simulink model "sm_import_stewart_platform"  (R2021b)
settings: Solver=ode45  StartTime=0.0  StopTime=10.0  RelTol=1e-3  EnableMultiTasking=on
model workspace (MATLAB code in the model file):
  | % The six origin vectors correspond to the six legs of the Stewart platform
  | stewart_pos_base = [0.0962 0 -0.0336; 0.0772 0 -0.0665;-0.0742 0 -0.0599;...
  |     -0.0962 0 -0.0336; -0.0190 0 0.1001;0.019 0 0.1001];
  | 
  | % Corresponding body points on the top plate
  | stewart_body_pts = [0.0607 0 0.0203; 0.0128 0 -0.0628; -0.0145 0 -0.0669; ...
  |     -0.0652 0 0.0208; -0.0507 0 0.046; 0.0507 0 0.046]';
  | 
  | % Leg length
  | leg_length = 0.19*ones(1,6);
undefined symbols (not defined in the file): X, Y, Z
libraries: sm_lib x1374, nesl_utility x19
(part 16 of 28)

== system sm_import_stewart_platform/Stewart Platform/Imported Stewart Platform/ActuatorAssm1_2/CarrierAssm_1_RIGID/HR_1_Motor_1_RIGID ==
  ReferenceFrame : sm_lib/Frames and Transforms/Reference Frame
  Solid : sm_lib/Body Elements/File Solid  ExtGeomFileName=HR_1_Motor_Default_sldprt.STL  UnitType=Custom  ExtGeomFileUnits=cm  StepReaderType=HEX  ExportConvexHullGeometry=off  InertiaType=Custom  Mass=0.016323277951690116  MassUnits=kg  CenterOfMass=[1.1461762495150611 1.9087990143138187 0.39999826480475109]  CenterOfMassUnits=cm  MomentsOfInertia=[0.022976248526302246 0.016967187564536409 0.038272540312041692]  MomentsOfInertiaUnits=kg*cm^2  ProductsOfInertia=[-6.3449814973716521e-08 -1.4415405966206584e-07 -0.0031628803180496112]  ProductsOfInertiaUnits=kg*cm^2  BasedOnType=Density  Density=1000  DensityUnits=kg/(m^3)  DoExposeReferenceFrame=on  SerializedFrames=<Frames/>  GraphicType=FromGeometry  MarkerShape=Sphere  MarkerSize=10  MarkerSizeUnits=m  GraphicVisPropType=SimpleVisualProperties  GraphicDiffuseColor=[0.95999999999999996 0.69647058823529406 0.56847058823529406]  GraphicSpecularColor=[0.5 0.5 0.5 1.0]  GraphicAmbientColor=[0.15 0.15 0.15 1.0]  GraphicEmissiveColor=[0.0 0.0 0.0 1.0]  GraphicShininess=75  GraphicOpacity=1
  F : PMIOPort  Side=Left
  connections:
  ReferenceFrame/RConn1 -- Solid/RConn1 -- F/RConn1

== system sm_import_stewart_platform/Stewart Platform/Imported Stewart Platform/ActuatorAssm1_2/CarrierAssm_1_RIGID/HR_1_Motor_2_RIGID ==
  ReferenceFrame : sm_lib/Frames and Transforms/Reference Frame
  Solid : sm_lib/Body Elements/File Solid  ExtGeomFileName=HR_1_Motor_Default_sldprt.STL  UnitType=Custom  ExtGeomFileUnits=cm  StepReaderType=HEX  ExportConvexHullGeometry=off  InertiaType=Custom  Mass=0.016323277951690116  MassUnits=kg  CenterOfMass=[1.1461762495150611 1.9087990143138187 0.39999826480475109]  CenterOfMassUnits=cm  MomentsOfInertia=[0.022976248526302246 0.016967187564536409 0.038272540312041692]  MomentsOfInertiaUnits=kg*cm^2  ProductsOfInertia=[-6.3449814973716521e-08 -1.4415405966206584e-07 -0.0031628803180496112]  ProductsOfInertiaUnits=kg*cm^2  BasedOnType=Density  Density=1000  DensityUnits=kg/(m^3)  DoExposeReferenceFrame=on  SerializedFrames=<Frames/>  GraphicType=FromGeometry  MarkerShape=Sphere  MarkerSize=10  MarkerSizeUnits=m  GraphicVisPropType=SimpleVisualProperties  GraphicDiffuseColor=[0.95999999999999996 0.69647058823529406 0.56847058823529406]  GraphicSpecularColor=[0.5 0.5 0.5 1.0]  GraphicAmbientColor=[0.15 0.15 0.15 1.0]  GraphicEmissiveColor=[0.0 0.0 0.0 1.0]  GraphicShininess=75  GraphicOpacity=1
  F : PMIOPort  Side=Left
  connections:
  ReferenceFrame/RConn1 -- Solid/RConn1 -- F/RConn1

== system sm_import_stewart_platform/Stewart Platform/Imported Stewart Platform/ActuatorAssm1_2/CarrierAssm_1_RIGID/Hexagon_Socket_Button_Head_Screw_M3x6_1_RIGID ==
  ReferenceFrame : sm_lib/Frames and Transforms/Reference Frame
  Solid : sm_lib/Body Elements/File Solid  ExtGeomFileName=Hexagon_Socket_Button_Head_Screw_M3x6_Default_sldprt.STL  UnitType=Custom  ExtGeomFileUnits=cm  StepReaderType=HEX  ExportConvexHullGeometry=off  InertiaType=Custom  Mass=0.00056348185373580135  MassUnits=kg  CenterOfMass=[0.14356282026314221 8.1476592298985412e-06 5.8788316934839061e-08]  CenterOfMassUnits=cm  MomentsOfInertia=[1.3098988700385332e-05 3.5078394083955334e-05 3.5077439490752727e-05]  MomentsOfInertiaUnits=kg*cm^2  ProductsOfInertia=[-6.7519077190030419e-11 7.6873810692743504e-12 1.0654186206953444e-09]  ProductsOfInertiaUnits=kg*cm^2  BasedOnType=Density  Density=1000  DensityUnits=kg/(m^3)  DoExposeReferenceFrame=on  SerializedFrames=<Frames/>  GraphicType=FromGeometry  MarkerShape=Sphere  MarkerSize=10  MarkerSizeUnits=m  GraphicVisPropType=SimpleVisualProperties  GraphicDiffuseColor=[0.72282352941176464 0.72282352941176464 0.72282352941176464]  GraphicSpecularColor=[0.5 0.5 0.5 1.0]  GraphicAmbientColor=[0.15 0.15 0.15 1.0]  GraphicEmissiveColor=[0.0 0.0 0.0 1.0]  GraphicShininess=75  GraphicOpacity=1
  F : PMIOPort  Side=Left
  connections:
  ReferenceFrame/RConn1 -- Solid/RConn1 -- F/RConn1

== system sm_import_stewart_platform/Stewart Platform/Imported Stewart Platform/ActuatorAssm1_2/CarrierAssm_1_RIGID/Hexagon_Socket_Button_Head_Screw_M3x6_2_RIGID ==
  ReferenceFrame : sm_lib/Frames and Transforms/Reference Frame
  Solid : sm_lib/Body Elements/File Solid  ExtGeomFileName=Hexagon_Socket_Button_Head_Screw_M3x6_Default_sldprt.STL  UnitType=Custom  ExtGeomFileUnits=cm  StepReaderType=HEX  ExportConvexHullGeometry=off  InertiaType=Custom  Mass=0.00056348185373580135  MassUnits=kg  CenterOfMass=[0.14356282026314221 8.1476592298985412e-06 5.8788316934839061e-08]  CenterOfMassUnits=cm  MomentsOfInertia=[1.3098988700385332e-05 3.5078394083955334e-05 3.5077439490752727e-05]  MomentsOfInertiaUnits=kg*cm^2  ProductsOfInertia=[-6.7519077190030419e-11 7.6873810692743504e-12 1.0654186206953444e-09]  ProductsOfInertiaUnits=kg*cm^2  BasedOnType=Density  Density=1000  DensityUnits=kg/(m^3)  DoExposeReferenceFrame=on  SerializedFrames=<Frames/>  GraphicType=FromGeometry  MarkerShape=Sphere  MarkerSize=10  MarkerSizeUnits=m  GraphicVisPropType=SimpleVisualProperties  GraphicDiffuseColor=[0.72282352941176464 0.72282352941176464 0.72282352941176464]  GraphicSpecularColor=[0.5 0.5 0.5 1.0]  GraphicAmbientColor=[0.15 0.15 0.15 1.0]  GraphicEmissiveColor=[0.0 0.0 0.0 1.0]  GraphicShininess=75  GraphicOpacity=1
  F : PMIOPort  Side=Left
  connections:
  ReferenceFrame/RConn1 -- Solid/RConn1 -- F/RConn1

== system sm_import_stewart_platform/Stewart Platform/Imported Stewart Platform/ActuatorAssm1_2/CarrierAssm_1_RIGID/Hexagon_Socket_Button_Head_Screw_M3x6_3_RIGID ==
  ReferenceFrame : sm_lib/Frames and Transforms/Reference Frame
  Solid : sm_lib/Body Elements/File Solid  ExtGeomFileName=Hexagon_Socket_Button_Head_Screw_M3x6_Default_sldprt.STL  UnitType=Custom  ExtGeomFileUnits=cm  StepReaderType=HEX  ExportConvexHullGeometry=off  InertiaType=Custom  Mass=0.00056348185373580135  MassUnits=kg  CenterOfMass=[0.14356282026314221 8.1476592298985412e-06 5.8788316934839061e-08]  CenterOfMassUnits=cm  MomentsOfInertia=[1.3098988700385332e-05 3.5078394083955334e-05 3.5077439490752727e-05]  MomentsOfInertiaUnits=kg*cm^2  ProductsOfInertia=[-6.7519077190030419e-11 7.6873810692743504e-12 1.0654186206953444e-09]  ProductsOfInertiaUnits=kg*cm^2  BasedOnType=Density  Density=1000  DensityUnits=kg/(m^3)  DoExposeReferenceFrame=on  SerializedFrames=<Frames/>  GraphicType=FromGeometry  MarkerShape=Sphere  MarkerSize=10  MarkerSizeUnits=m  GraphicVisPropType=SimpleVisualProperties  GraphicDiffuseColor=[0.72282352941176464 0.72282352941176464 0.72282352941176464]  GraphicSpecularColor=[0.5 0.5 0.5 1.0]  GraphicAmbientColor=[0.15 0.15 0.15 1.0]  GraphicEmissiveColor=[0.0 0.0 0.0 1.0]  GraphicShininess=75  GraphicOpacity=1
  F : PMIOPort  Side=Left
  connections:
  ReferenceFrame/RConn1 -- Solid/RConn1 -- F/RConn1

== system sm_import_stewart_platform/Stewart Platform/Imported Stewart Platform/ActuatorAssm1_2/CarrierAssm_1_RIGID/Hexagon_Socket_Button_Head_Screw_M3x6_4_RIGID ==
  ReferenceFrame : sm_lib/Frames and Transforms/Reference Frame
  Solid : sm_lib/Body Elements/File Solid  ExtGeomFileName=Hexagon_Socket_Button_Head_Screw_M3x6_Default_sldprt.STL  UnitType=Custom  ExtGeomFileUnits=cm  StepReaderType=HEX  ExportConvexHullGeometry=off  InertiaType=Custom  Mass=0.00056348185373580135  MassUnits=kg  CenterOfMass=[0.14356282026314221 8.1476592298985412e-06 5.8788316934839061e-08]  CenterOfMassUnits=cm  MomentsOfInertia=[1.3098988700385332e-05 3.5078394083955334e-05 3.5077439490752727e-05]  MomentsOfInertiaUnits=kg*cm^2  ProductsOfInertia=[-6.7519077190030419e-11 7.6873810692743504e-12 1.0654186206953444e-09]  ProductsOfInertiaUnits=kg*cm^2  BasedOnType=Density  Density=1000  DensityUnits=kg/(m^3)  DoExposeReferenceFrame=on  SerializedFrames=<Frames/>  GraphicType=FromGeometry  MarkerShape=Sphere  MarkerSize=10  MarkerSizeUnits=m  GraphicVisPropType=SimpleVisualProperties  GraphicDiffuseColor=[0.72282352941176464 0.72282352941176464 0.72282352941176464]  GraphicSpecularColor=[0.5 0.5 0.5 1.0]  GraphicAmbientColor=[0.15 0.15 0.15 1.0]  GraphicEmissiveColor=[0.0 0.0 0.0 1.0]  GraphicShininess=75  GraphicOpacity=1
  F : PMIOPort  Side=Left
  connections:
  ReferenceFrame/RConn1 -- Solid/RConn1 -- F/RConn1

== system sm_import_stewart_platform/Stewart Platform/Imported Stewart Platform/ActuatorAssm1_2/CarrierAssm_1_RIGID/Hexagon_Socket_Button_Head_Screw_M3x6_5_RIGID ==
  ReferenceFrame : sm_lib/Frames and Transforms/Reference Frame
  Solid : sm_lib/Body Elements/File Solid  ExtGeomFileName=Hexagon_Socket_Button_Head_Screw_M3x6_Default_sldprt.STL  UnitType=Custom  ExtGeomFileUnits=cm  StepReaderType=HEX  ExportConvexHullGeometry=off  InertiaType=Custom  Mass=0.00056348185373580135  MassUnits=kg  CenterOfMass=[0.14356282026314221 8.1476592298985412e-06 5.8788316934839061e-08]  CenterOfMassUnits=cm  MomentsOfInertia=[1.3098988700385332e-05 3.5078394083955334e-05 3.5077439490752727e-05]  MomentsOfInertiaUnits=kg*cm^2  ProductsOfInertia=[-6.7519077190030419e-11 7.6873810692743504e-12 1.0654186206953444e-09]  ProductsOfInertiaUnits=kg*cm^2  BasedOnType=Density  Density=1000  DensityUnits=kg/(m^3)  DoExposeReferenceFrame=on  SerializedFrames=<Frames/>  GraphicType=FromGeometry  MarkerShape=Sphere  MarkerSize=10  MarkerSizeUnits=m  GraphicVisPropType=SimpleVisualProperties  GraphicDiffuseColor=[0.72282352941176464 0.72282352941176464 0.72282352941176464]  GraphicSpecularColor=[0.5 0.5 0.5 1.0]  GraphicAmbientColor=[0.15 0.15 0.15 1.0]  GraphicEmissiveColor=[0.0 0.0 0.0 1.0]  GraphicShininess=75  GraphicOpacity=1
  F : PMIOPort  Side=Left
  connections:
  ReferenceFrame/RConn1 -- Solid/RConn1 -- F/RConn1

== system sm_import_stewart_platform/Stewart Platform/Imported Stewart Platform/ActuatorAssm1_2/CarrierAssm_1_RIGID/Hexagon_Socket_Button_Head_Screw_M3x6_6_RIGID ==
  ReferenceFrame : sm_lib/Frames and Transforms/Reference Frame
  Solid : sm_lib/Body Elements/File Solid  ExtGeomFileName=Hexagon_Socket_Button_Head_Screw_M3x6_Default_sldprt.STL  UnitType=Custom  ExtGeomFileUnits=cm  StepReaderType=HEX  ExportConvexHullGeometry=off  InertiaType=Custom  Mass=0.00056348185373580135  MassUnits=kg  CenterOfMass=[0.14356282026314221 8.1476592298985412e-06 5.8788316934839061e-08]  CenterOfMassUnits=cm  MomentsOfInertia=[1.3098988700385332e-05 3.5078394083955334e-05 3.5077439490752727e-05]  MomentsOfInertiaUnits=kg*cm^2  ProductsOfInertia=[-6.7519077190030419e-11 7.6873810692743504e-12 1.0654186206953444e-09]  ProductsOfInertiaUnits=kg*cm^2  BasedOnType=Density  Density=1000  DensityUnits=kg/(m^3)  DoExposeReferenceFrame=on  SerializedFrames=<Frames/>  GraphicType=FromGeometry  MarkerShape=Sphere  MarkerSize=10  MarkerSizeUnits=m  GraphicVisPropType=SimpleVisualProperties  GraphicDiffuseColor=[0.72282352941176464 0.72282352941176464 0.72282352941176464]  GraphicSpecularColor=[0.5 0.5 0.5 1.0]  GraphicAmbientColor=[0.15 0.15 0.15 1.0]  GraphicEmissiveColor=[0.0 0.0 0.0 1.0]  GraphicShininess=75  GraphicOpacity=1
  F : PMIOPort  Side=Left
  connections:
  ReferenceFrame/RConn1 -- Solid/RConn1 -- F/RConn1

== system sm_import_stewart_platform/Stewart Platform/Imported Stewart Platform/ActuatorAssm1_2/CarrierAssm_1_RIGID/Hexagon_Socket_Button_Head_Screw_M3x6_7_RIGID ==
  ReferenceFrame : sm_lib/Frames and Transforms/Reference Frame
  Solid : sm_lib/Body Elements/File Solid  ExtGeomFileName=Hexagon_Socket_Button_Head_Screw_M3x6_Default_sldprt.STL  UnitType=Custom  ExtGeomFileUnits=cm  StepReaderType=HEX  ExportConvexHullGeometry=off  InertiaType=Custom  Mass=0.00056348185373580135  MassUnits=kg  CenterOfMass=[0.14356282026314221 8.1476592298985412e-06 5.8788316934839061e-08]  CenterOfMassUnits=cm  MomentsOfInertia=[1.3098988700385332e-05 3.5078394083955334e-05 3.5077439490752727e-05]  MomentsOfInertiaUnits=kg*cm^2  ProductsOfInertia=[-6.7519077190030419e-11 7.6873810692743504e-12 1.0654186206953444e-09]  ProductsOfInertiaUnits=kg*cm^2  BasedOnType=Density  Density=1000  DensityUnits=kg/(m^3)  DoExposeReferenceFrame=on  SerializedFrames=<Frames/>  GraphicType=FromGeometry  MarkerShape=Sphere  MarkerSize=10  MarkerSizeUnits=m  GraphicVisPropType=SimpleVisualProperties  GraphicDiffuseColor=[0.72282352941176464 0.72282352941176464 0.72282352941176464]  GraphicSpecularColor=[0.5 0.5 0.5 1.0]  GraphicAmbientColor=[0.15 0.15 0.15 1.0]  GraphicEmissiveColor=[0.0 0.0 0.0 1.0]  GraphicShininess=75  GraphicOpacity=1
  F : PMIOPort  Side=Left
  connections:
  ReferenceFrame/RConn1 -- Solid/RConn1 -- F/RConn1

== system sm_import_stewart_platform/Stewart Platform/Imported Stewart Platform/ActuatorAssm1_2/CarrierAssm_1_RIGID/Hexagon_Socket_Button_Head_Screw_M3x6_8_RIGID ==
  ReferenceFrame : sm_lib/Frames and Transforms/Reference Frame
  Solid : sm_lib/Body Elements/File Solid  ExtGeomFileName=Hexagon_Socket_Button_Head_Screw_M3x6_Default_sldprt.STL  UnitType=Custom  ExtGeomFileUnits=cm  StepReaderType=HEX  ExportConvexHullGeometry=off  InertiaType=Custom  Mass=0.00056348185373580135  MassUnits=kg  CenterOfMass=[0.14356282026314221 8.1476592298985412e-06 5.8788316934839061e-08]  CenterOfMassUnits=cm  MomentsOfInertia=[1.3098988700385332e-05 3.5078394083955334e-05 3.5077439490752727e-05]  MomentsOfInertiaUnits=kg*cm^2  ProductsOfInertia=[-6.7519077190030419e-11 7.6873810692743504e-12 1.0654186206953444e-09]  ProductsOfInertiaUnits=kg*cm^2  BasedOnType=Density  Density=1000  DensityUnits=kg/(m^3)  DoExposeReferenceFrame=on  SerializedFrames=<Frames/>  GraphicType=FromGeometry  MarkerShape=Sphere  MarkerSize=10  MarkerSizeUnits=m  GraphicVisPropType=SimpleVisualProperties  GraphicDiffuseColor=[0.72282352941176464 0.72282352941176464 0.72282352941176464]  GraphicSpecularColor=[0.5 0.5 0.5 1.0]  GraphicAmbientColor=[0.15 0.15 0.15 1.0]  GraphicEmissiveColor=[0.0 0.0 0.0 1.0]  GraphicShininess=75  GraphicOpacity=1
  F : PMIOPort  Side=Left
  connections:
  ReferenceFrame/RConn1 -- Solid/RConn1 -- F/RConn1

== system sm_import_stewart_platform/Stewart Platform/Imported Stewart Platform/ActuatorAssm1_2/CarrierAssm_1_RIGID/Hexagon_Socket_Head_Cap_Screw_M3x5_1_RIGID ==
  ReferenceFrame : sm_lib/Frames and Transforms/Reference Frame
  Solid : sm_lib/Body Elements/File Solid  ExtGeomFileName=Hexagon_Socket_Head_Cap_Screw_M3x5_Default_sldprt.STL  UnitType=Custom  ExtGeomFileUnits=cm  StepReaderType=HEX  ExportConvexHullGeometry=off  InertiaType=Custom  Mass=0.00075563833672042757  MassUnits=kg  CenterOfMass=[-0.00070356125816108312 3.3976681789998727e-05 2.4288939549848704e-07]  CenterOfMassUnits=cm  MomentsOfInertia=[2.3283103549749918e-05 4.6860987295278262e-05 4.6851281632327237e-05]  MomentsOfInertiaUnits=kg*cm^2  ProductsOfInertia=[-6.6364273820729613e-10 4.0249100574764394e-11 5.6302615064034264e-09]  ProductsOfInertiaUnits=kg*cm^2  BasedOnType=Density  Density=1000  DensityUnits=kg/(m^3)  DoExposeReferenceFrame=on  SerializedFrames=<Frames/>  GraphicType=FromGeometry  MarkerShape=Sphere  MarkerSize=10  MarkerSizeUnits=m  GraphicVisPropType=SimpleVisualProperties  GraphicDiffuseColor=[0.72282352941176464 0.72282352941176464 0.72282352941176464]  GraphicSpecularColor=[0.5 0.5 0.5 1.0]  GraphicAmbientColor=[0.15 0.15 0.15 1.0]  GraphicEmissiveColor=[0.0 0.0 0.0 1.0]  GraphicShininess=75  GraphicOpacity=1
  F : PMIOPort  Side=Left
  connections:
  ReferenceFrame/RConn1 -- Solid/RConn1 -- F/RConn1

== system sm_import_stewart_platform/Stewart Platform/Imported Stewart Platform/ActuatorAssm1_2/CarrierAssm_1_RIGID/Hexagon_Socket_Head_Cap_Screw_M3x5_2_RIGID ==
  ReferenceFrame : sm_lib/Frames and Transforms/Reference Frame
  Solid : sm_lib/Body Elements/File Solid  ExtGeomFileName=Hexagon_Socket_Head_Cap_Screw_M3x5_Default_sldprt.STL  UnitType=Custom  ExtGeomFileUnits=cm  StepReaderType=HEX  ExportConvexHullGeometry=off  InertiaType=Custom  Mass=0.00075563833672042757  MassUnits=kg  CenterOfMass=[-0.00070356125816108312 3.3976681789998727e-05 2.4288939549848704e-07]  CenterOfMassUnits=cm  MomentsOfInertia=[2.3283103549749918e-05 4.6860987295278262e-05 4.6851281632327237e-05]  MomentsOfInertiaUnits=kg*cm^2  ProductsOfInertia=[-6.6364273820729613e-10 4.0249100574764394e-11 5.6302615064034264e-09]  ProductsOfInertiaUnits=kg*cm^2  BasedOnType=Density  Density=1000  DensityUnits=kg/(m^3)  DoExposeReferenceFrame=on  SerializedFrames=<Frames/>  GraphicType=FromGeometry  MarkerShape=Sphere  MarkerSize=10  MarkerSizeUnits=m  GraphicVisPropType=SimpleVisualProperties  GraphicDiffuseColor=[0.72282352941176464 0.72282352941176464 0.72282352941176464]  GraphicSpecularColor=[0.5 0.5 0.5 1.0]  GraphicAmbientColor=[0.15 0.15 0.15 1.0]  GraphicEmissiveColor=[0.0 0.0 0.0 1.0]  GraphicShininess=75  GraphicOpacity=1
  F : PMIOPort  Side=Left
  connections:
  ReferenceFrame/RConn1 -- Solid/RConn1 -- F/RConn1

== system sm_import_stewart_platform/Stewart Platform/Imported Stewart Platform/ActuatorAssm1_2/CarrierAssm_1_RIGID/Hexagon_Socket_Set_Screw_M3x3_1_RIGID ==
  ReferenceFrame : sm_lib/Frames and Transforms/Reference Frame
  Solid : sm_lib/Body Elements/File Solid  ExtGeomFileName=Hexagon_Socket_Set_Screw_M3x3_Default_sldprt.STL  UnitType=Custom  ExtGeomFileUnits=cm  StepReaderType=HEX  ExportConvexHullGeometry=off  InertiaType=Custom  Mass=0.00013414962639699338  MassUnits=kg  CenterOfMass=[0.14346797240988166 0 0]  CenterOfMassUnits=cm  MomentsOfInertia=[1.6122422751910497e-06 1.6862757603444589e-06 1.6862757577761036e-06]  MomentsOfInertiaUnits=kg*cm^2  ProductsOfInertia=[0 0 0]  ProductsOfInertiaUnits=kg*cm^2  BasedOnType=Density  Density=1000  DensityUnits=kg/(m^3)  DoExposeReferenceFrame=on  SerializedFrames=<Frames/>  GraphicType=FromGeometry  MarkerShape=Sphere  MarkerSize=10  MarkerSizeUnits=m  GraphicVisPropType=SimpleVisualProperties  GraphicDiffuseColor=[0.72282352941176464 0.72282352941176464 0.72282352941176464]  GraphicSpecularColor=[0.5 0.5 0.5 1.0]  GraphicAmbientColor=[0.15 0.15 0.15 1.0]  GraphicEmissiveColor=[0.0 0.0 0.0 1.0]  GraphicShininess=75  GraphicOpacity=1
  F : PMIOPort  Side=Left
  connections:
  ReferenceFrame/RConn1 -- Solid/RConn1 -- F/RConn1

== system sm_import_stewart_platform/Stewart Platform/Imported Stewart Platform/ActuatorAssm1_2/CarrierAssm_1_RIGID/Hexagon_Socket_Set_Screw_M3x3_2_RIGID ==
  ReferenceFrame : sm_lib/Frames and Transforms/Reference Frame
  Solid : sm_lib/Body Elements/File Solid  ExtGeomFileName=Hexagon_Socket_Set_Screw_M3x3_Default_sldprt.STL  UnitType=Custom  ExtGeomFileUnits=cm  StepReaderType=HEX  ExportConvexHullGeometry=off  InertiaType=Custom  Mass=0.00013414962639699338  MassUnits=kg  CenterOfMass=[0.14346797240988166 0 0]  CenterOfMassUnits=cm  MomentsOfInertia=[1.6122422751910497e-06 1.6862757603444589e-06 1.6862757577761036e-06]  MomentsOfInertiaUnits=kg*cm^2  ProductsOfInertia=[0 0 0]  ProductsOfInertiaUnits=kg*cm^2  BasedOnType=Density  Density=1000  DensityUnits=kg/(m^3)  DoExposeReferenceFrame=on  SerializedFrames=<Frames/>  GraphicType=FromGeometry  MarkerShape=Sphere  MarkerSize=10  MarkerSizeUnits=m  GraphicVisPropType=SimpleVisualProperties  GraphicDiffuseColor=[0.72282352941176464 0.72282352941176464 0.72282352941176464]  GraphicSpecularColor=[0.5 0.5 0.5 1.0]  GraphicAmbientColor=[0.15 0.15 0.15 1.0]  GraphicEmissiveColor=[0.0 0.0 0.0 1.0]  GraphicShininess=75  GraphicOpacity=1
  F : PMIOPort  Side=Left
  connections:
  ReferenceFrame/RConn1 -- Solid/RConn1 -- F/RConn1

== system sm_import_stewart_platform/Stewart Platform/Imported Stewart Platform/ActuatorAssm1_2/CarrierAssm_1_RIGID/Hexagon_Socket_Set_Screw_M3x3_3_RIGID ==
  ReferenceFrame : sm_lib/Frames and Transforms/Reference Frame
  Solid : sm_lib/Body Elements/File Solid  ExtGeomFileName=Hexagon_Socket_Set_Screw_M3x3_Default_sldprt.STL  UnitType=Custom  ExtGeomFileUnits=cm  StepReaderType=HEX  ExportConvexHullGeometry=off  InertiaType=Custom  Mass=0.00013414962639699338  MassUnits=kg  CenterOfMass=[0.14346797240988166 0 0]  CenterOfMassUnits=cm  MomentsOfInertia=[1.6122422751910497e-06 1.6862757603444589e-06 1.6862757577761036e-06]  MomentsOfInertiaUnits=kg*cm^2  ProductsOfInertia=[0 0 0]  ProductsOfInertiaUnits=kg*cm^2  BasedOnType=Density  Density=1000  DensityUnits=kg/(m^3)  DoExposeReferenceFrame=on  SerializedFrames=<Frames/>  GraphicType=FromGeometry  MarkerShape=Sphere  MarkerSize=10  MarkerSizeUnits=m  GraphicVisPropType=SimpleVisualProperties  GraphicDiffuseColor=[0.72282352941176464 0.72282352941176464 0.72282352941176464]  GraphicSpecularColor=[0.5 0.5 0.5 1.0]  GraphicAmbientColor=[0.15 0.15 0.15 1.0]  GraphicEmissiveColor=[0.0 0.0 0.0 1.0]  GraphicShininess=75  GraphicOpacity=1
  F : PMIOPort  Side=Left
  connections:
  ReferenceFrame/RConn1 -- Solid/RConn1 -- F/RConn1

== system sm_import_stewart_platform/Stewart Platform/Imported Stewart Platform/ActuatorAssm1_2/CarrierAssm_1_RIGID/Hexagon_Socket_Set_Screw_M3x3_4_RIGID ==
  ReferenceFrame : sm_lib/Frames and Transforms/Reference Frame
  Solid : sm_lib/Body Elements/File Solid  ExtGeomFileName=Hexagon_Socket_Set_Screw_M3x3_Default_sldprt.STL  UnitType=Custom  ExtGeomFileUnits=cm  StepReaderType=HEX  ExportConvexHullGeometry=off  InertiaType=Custom  Mass=0.00013414962639699338  MassUnits=kg  CenterOfMass=[0.14346797240988166 0 0]  CenterOfMassUnits=cm  MomentsOfInertia=[1.6122422751910497e-06 1.6862757603444589e-06 1.6862757577761036e-06]  MomentsOfInertiaUnits=kg*cm^2  ProductsOfInertia=[0 0 0]  ProductsOfInertiaUnits=kg*cm^2  BasedOnType=Density  Density=1000  DensityUnits=kg/(m^3)  DoExposeReferenceFrame=on  SerializedFrames=<Frames/>  GraphicType=FromGeometry  MarkerShape=Sphere  MarkerSize=10  MarkerSizeUnits=m  GraphicVisPropType=SimpleVisualProperties  GraphicDiffuseColor=[0.72282352941176464 0.72282352941176464 0.72282352941176464]  GraphicSpecularColor=[0.5 0.5 0.5 1.0]  GraphicAmbientColor=[0.15 0.15 0.15 1.0]  GraphicEmissiveColor=[0.0 0.0 0.0 1.0]  GraphicShininess=75  GraphicOpacity=1
  F : PMIOPort  Side=Left
  connections:
  ReferenceFrame/RConn1 -- Solid/RConn1 -- F/RConn1

== system sm_import_stewart_platform/Stewart Platform/Imported Stewart Platform/ActuatorAssm1_2/CarrierAssm_1_RIGID/Hexagon_Socket_Set_Screw_M3x3_5_RIGID ==
  ReferenceFrame : sm_lib/Frames and Transforms/Reference Frame
  Solid : sm_lib/Body Elements/File Solid  ExtGeomFileName=Hexagon_Socket_Set_Screw_M3x3_Default_sldprt.STL  UnitType=Custom  ExtGeomFileUnits=cm  StepReaderType=HEX  ExportConvexHullGeometry=off  InertiaType=Custom  Mass=0.00013414962639699338  MassUnits=kg  CenterOfMass=[0.14346797240988166 0 0]  CenterOfMassUnits=cm  MomentsOfInertia=[1.6122422751910497e-06 1.6862757603444589e-06 1.6862757577761036e-06]  MomentsOfInertiaUnits=kg*cm^2  ProductsOfInertia=[0 0 0]  ProductsOfInertiaUnits=kg*cm^2  BasedOnType=Density  Density=1000  DensityUnits=kg/(m^3)  DoExposeReferenceFrame=on  SerializedFrames=<Frames/>  GraphicType=FromGeometry  MarkerShape=Sphere  MarkerSize=10  MarkerSizeUnits=m  GraphicVisPropType=SimpleVisualProperties  GraphicDiffuseColor=[0.72282352941176464 0.72282352941176464 0.72282352941176464]  GraphicSpecularColor=[0.5 0.5 0.5 1.0]  GraphicAmbientColor=[0.15 0.15 0.15 1.0]  GraphicEmissiveColor=[0.0 0.0 0.0 1.0]  GraphicShininess=75  GraphicOpacity=1
  F : PMIOPort  Side=Left
  connections:
  ReferenceFrame/RConn1 -- Solid/RConn1 -- F/RConn1

== system sm_import_stewart_platform/Stewart Platform/Imported Stewart Platform/ActuatorAssm1_2/CarrierAssm_1_RIGID/RGH25_1_RIGID ==
  ReferenceFrame : sm_lib/Frames and Transforms/Reference Frame
  Solid : sm_lib/Body Elements/File Solid  ExtGeomFileName=RGH25_Default_sldprt.STL  UnitType=Custom  ExtGeomFileUnits=cm  StepReaderType=HEX  ExportConvexHullGeometry=off  InertiaType=Custom  Mass=0.01179296125695376  MassUnits=kg  CenterOfMass=[0.23437231077884074 0.044553543526049413 0.96324975911409805]  CenterOfMassUnits=cm  MomentsOfInertia=[0.056374702857213979 0.060512471256549662 0.0060033931898553225]  MomentsOfInertiaUnits=kg*cm^2  ProductsOfInertia=[0.0011970125178576842 0.011872429161589867 -0.00034145940679604055]  ProductsOfInertiaUnits=kg*cm^2  BasedOnType=Density  Density=1000  DensityUnits=kg/(m^3)  DoExposeReferenceFrame=on  SerializedFrames=<Frames/>  GraphicType=FromGeometry  MarkerShape=Sphere  MarkerSize=10  MarkerSizeUnits=m  GraphicVisPropType=SimpleVisualProperties  GraphicDiffuseColor=[0.59105882352941175 0.95999999999999996 0.59105882352941175]  GraphicSpecularColor=[0.5 0.5 0.5 1.0]  GraphicAmbientColor=[0.15 0.15 0.15 1.0]  GraphicEmissiveColor=[0.0 0.0 0.0 1.0]  GraphicShininess=75  GraphicOpacity=1
  F : PMIOPort  Side=Left
  connections:
  ReferenceFrame/RConn1 -- Solid/RConn1 -- F/RConn1

== system sm_import_stewart_platform/Stewart Platform/Imported Stewart Platform/ActuatorAssm1_2/CarrierAssm_1_RIGID/Recessed_Pan_Head_Screw_M2x8_48_Z_10_RIGID ==
  ReferenceFrame : sm_lib/Frames and Transforms/Reference Frame
  Solid : sm_lib/Body Elements/File Solid  ExtGeomFileName=Recessed_Pan_Head_Screw_M2x8_48_Z_Default_sldprt.STL  UnitType=Custom  ExtGeomFileUnits=cm  StepReaderType=HEX  ExportConvexHullGeometry=off  InertiaType=Custom  Mass=0.00030420054001085506  MassUnits=kg  CenterOfMass=[0.23057963245570592 -4.2158298307861626e-10 -1.6472469656016965e-11]  CenterOfMassUnits=cm  MomentsOfInertia=[3.0541038740142581e-06 2.6916548970402947e-05 2.6916548962268568e-05]  MomentsOfInertiaUnits=kg*cm^2  ProductsOfInertia=[0 0 0]  ProductsOfInertiaUnits=kg*cm^2  BasedOnType=Density  Density=1000  DensityUnits=kg/(m^3)  DoExposeReferenceFrame=on  SerializedFrames=<Frames/>  GraphicType=FromGeometry  MarkerShape=Sphere  MarkerSize=10  MarkerSizeUnits=m  GraphicVisPropType=SimpleVisualProperties  GraphicDiffuseColor=[0.72282352941176464 0.72282352941176464 0.72282352941176464]  GraphicSpecularColor=[0.5 0.5 0.5 1.0]  GraphicAmbientColor=[0.15 0.15 0.15 1.0]  GraphicEmissiveColor=[0.0 0.0 0.0 1.0]  GraphicShininess=75  GraphicOpacity=1
  F : PMIOPort  Side=Left
  connections:
  ReferenceFrame/RConn1 -- Solid/RConn1 -- F/RConn1

== system sm_import_stewart_platform/Stewart Platform/Imported Stewart Platform/ActuatorAssm1_2/CarrierAssm_1_RIGID/Recessed_Pan_Head_Screw_M2x8_48_Z_1_RIGID ==
  ReferenceFrame : sm_lib/Frames and Transforms/Reference Frame
  Solid : sm_lib/Body Elements/File Solid  ExtGeomFileName=Recessed_Pan_Head_Screw_M2x8_48_Z_Default_sldprt.STL  UnitType=Custom  ExtGeomFileUnits=cm  StepReaderType=HEX  ExportConvexHullGeometry=off  InertiaType=Custom  Mass=0.00030420054001085506  MassUnits=kg  CenterOfMass=[0.23057963245570592 -4.2158298307861626e-10 -1.6472469656016965e-11]  CenterOfMassUnits=cm  MomentsOfInertia=[3.0541038740142581e-06 2.6916548970402947e-05 2.6916548962268568e-05]  MomentsOfInertiaUnits=kg*cm^2  ProductsOfInertia=[0 0 0]  ProductsOfInertiaUnits=kg*cm^2  BasedOnType=Density  Density=1000  DensityUnits=kg/(m^3)  DoExposeReferenceFrame=on  SerializedFrames=<Frames/>  GraphicType=FromGeometry  MarkerShape=Sphere  MarkerSize=10  MarkerSizeUnits=m  GraphicVisPropType=SimpleVisualProperties  GraphicDiffuseColor=[0.72282352941176464 0.72282352941176464 0.72282352941176464]  GraphicSpecularColor=[0.5 0.5 0.5 1.0]  GraphicAmbientColor=[0.15 0.15 0.15 1.0]  GraphicEmissiveColor=[0.0 0.0 0.0 1.0]  GraphicShininess=75  GraphicOpacity=1
  F : PMIOPort  Side=Left
  connections:
  ReferenceFrame/RConn1 -- Solid/RConn1 -- F/RConn1

== system sm_import_stewart_platform/Stewart Platform/Imported Stewart Platform/ActuatorAssm1_2/CarrierAssm_1_RIGID/Recessed_Pan_Head_Screw_M2x8_48_Z_2_RIGID ==
  ReferenceFrame : sm_lib/Frames and Transforms/Reference Frame
  Solid : sm_lib/Body Elements/File Solid  ExtGeomFileName=Recessed_Pan_Head_Screw_M2x8_48_Z_Default_sldprt.STL  UnitType=Custom  ExtGeomFileUnits=cm  StepReaderType=HEX  ExportConvexHullGeometry=off  InertiaType=Custom  Mass=0.00030420054001085506  MassUnits=kg  CenterOfMass=[0.23057963245570592 -4.2158298307861626e-10 -1.6472469656016965e-11]  CenterOfMassUnits=cm  MomentsOfInertia=[3.0541038740142581e-06 2.6916548970402947e-05 2.6916548962268568e-05]  MomentsOfInertiaUnits=kg*cm^2  ProductsOfInertia=[0 0 0]  ProductsOfInertiaUnits=kg*cm^2  BasedOnType=Density  Density=1000  DensityUnits=kg/(m^3)  DoExposeReferenceFrame=on  SerializedFrames=<Frames/>  GraphicType=FromGeometry  MarkerShape=Sphere  MarkerSize=10  MarkerSizeUnits=m  GraphicVisPropType=SimpleVisualProperties  GraphicDiffuseColor=[0.72282352941176464 0.72282352941176464 0.72282352941176464]  GraphicSpecularColor=[0.5 0.5 0.5 1.0]  GraphicAmbientColor=[0.15 0.15 0.15 1.0]  GraphicEmissiveColor=[0.0 0.0 0.0 1.0]  GraphicShininess=75  GraphicOpacity=1
  F : PMIOPort  Side=Left
  connections:
  ReferenceFrame/RConn1 -- Solid/RConn1 -- F/RConn1

== system sm_import_stewart_platform/Stewart Platform/Imported Stewart Platform/ActuatorAssm1_2/CarrierAssm_1_RIGID/Recessed_Pan_Head_Screw_M2x8_48_Z_3_RIGID ==
  ReferenceFrame : sm_lib/Frames and Transforms/Reference Frame
  Solid : sm_lib/Body Elements/File Solid  ExtGeomFileName=Recessed_Pan_Head_Screw_M2x8_48_Z_Default_sldprt.STL  UnitType=Custom  ExtGeomFileUnits=cm  StepReaderType=HEX  ExportConvexHullGeometry=off  InertiaType=Custom  Mass=0.00030420054001085506  MassUnits=kg  CenterOfMass=[0.23057963245570592 -4.2158298307861626e-10 -1.6472469656016965e-11]  CenterOfMassUnits=cm  MomentsOfInertia=[3.0541038740142581e-06 2.6916548970402947e-05 2.6916548962268568e-05]  MomentsOfInertiaUnits=kg*cm^2  ProductsOfInertia=[0 0 0]  ProductsOfInertiaUnits=kg*cm^2  BasedOnType=Density  Density=1000  DensityUnits=kg/(m^3)  DoExposeReferenceFrame=on  SerializedFrames=<Frames/>  GraphicType=FromGeometry  MarkerShape=Sphere  MarkerSize=10  MarkerSizeUnits=m  GraphicVisPropType=SimpleVisualProperties  GraphicDiffuseColor=[0.72282352941176464 0.72282352941176464 0.72282352941176464]  GraphicSpecularColor=[0.5 0.5 0.5 1.0]  GraphicAmbientColor=[0.15 0.15 0.15 1.0]  GraphicEmissiveColor=[0.0 0.0 0.0 1.0]  GraphicShininess=75  GraphicOpacity=1
  F : PMIOPort  Side=Left
  connections:
  ReferenceFrame/RConn1 -- Solid/RConn1 -- F/RConn1

== system sm_import_stewart_platform/Stewart Platform/Imported Stewart Platform/ActuatorAssm1_2/CarrierAssm_1_RIGID/Recessed_Pan_Head_Screw_M2x8_48_Z_4_RIGID ==
  ReferenceFrame : sm_lib/Frames and Transforms/Reference Frame
  Solid : sm_lib/Body Elements/File Solid  ExtGeomFileName=Recessed_Pan_Head_Screw_M2x8_48_Z_Default_sldprt.STL  UnitType=Custom  ExtGeomFileUnits=cm  StepReaderType=HEX  ExportConvexHullGeometry=off  InertiaType=Custom  Mass=0.00030420054001085506  MassUnits=kg  CenterOfMass=[0.23057963245570592 -4.2158298307861626e-10 -1.6472469656016965e-11]  CenterOfMassUnits=cm  MomentsOfInertia=[3.0541038740142581e-06 2.6916548970402947e-05 2.6916548962268568e-05]  MomentsOfInertiaUnits=kg*cm^2  ProductsOfInertia=[0 0 0]  ProductsOfInertiaUnits=kg*cm^2  BasedOnType=Density  Density=1000  DensityUnits=kg/(m^3)  DoExposeReferenceFrame=on  SerializedFrames=<Frames/>  GraphicType=FromGeometry  MarkerShape=Sphere  MarkerSize=10  MarkerSizeUnits=m  GraphicVisPropType=SimpleVisualProperties  GraphicDiffuseColor=[0.72282352941176464 0.72282352941176464 0.72282352941176464]  GraphicSpecularColor=[0.5 0.5 0.5 1.0]  GraphicAmbientColor=[0.15 0.15 0.15 1.0]  GraphicEmissiveColor=[0.0 0.0 0.0 1.0]  GraphicShininess=75  GraphicOpacity=1
  F : PMIOPort  Side=Left
  connections:
  ReferenceFrame/RConn1 -- Solid/RConn1 -- F/RConn1

== system sm_import_stewart_platform/Stewart Platform/Imported Stewart Platform/ActuatorAssm1_2/CarrierAssm_1_RIGID/Recessed_Pan_Head_Screw_M2x8_48_Z_5_RIGID ==
  ReferenceFrame : sm_lib/Frames and Transforms/Reference Frame
  Solid : sm_lib/Body Elements/File Solid  ExtGeomFileName=Recessed_Pan_Head_Screw_M2x8_48_Z_Default_sldprt.STL  UnitType=Custom  ExtGeomFileUnits=cm  StepReaderType=HEX  ExportConvexHullGeometry=off  InertiaType=Custom  Mass=0.00030420054001085506  MassUnits=kg  CenterOfMass=[0.23057963245570592 -4.2158298307861626e-10 -1.6472469656016965e-11]  CenterOfMassUnits=cm  MomentsOfInertia=[3.0541038740142581e-06 2.6916548970402947e-05 2.6916548962268568e-05]  MomentsOfInertiaUnits=kg*cm^2  ProductsOfInertia=[0 0 0]  ProductsOfInertiaUnits=kg*cm^2  BasedOnType=Density  Density=1000  DensityUnits=kg/(m^3)  DoExposeReferenceFrame=on  SerializedFrames=<Frames/>  GraphicType=FromGeometry  MarkerShape=Sphere  MarkerSize=10  MarkerSizeUnits=m  GraphicVisPropType=SimpleVisualProperties  GraphicDiffuseColor=[0.72282352941176464 0.72282352941176464 0.72282352941176464]  GraphicSpecularColor=[0.5 0.5 0.5 1.0]  GraphicAmbientColor=[0.15 0.15 0.15 1.0]  GraphicEmissiveColor=[0.0 0.0 0.0 1.0]  GraphicShininess=75  GraphicOpacity=1
  F : PMIOPort  Side=Left
  connections:
  ReferenceFrame/RConn1 -- Solid/RConn1 -- F/RConn1

== system sm_import_stewart_platform/Stewart Platform/Imported Stewart Platform/ActuatorAssm1_2/CarrierAssm_1_RIGID/Recessed_Pan_Head_Screw_M2x8_48_Z_6_RIGID ==
  ReferenceFrame : sm_lib/Frames and Transforms/Reference Frame
  Solid : sm_lib/Body Elements/File Solid  ExtGeomFileName=Recessed_Pan_Head_Screw_M2x8_48_Z_Default_sldprt.STL  UnitType=Custom  ExtGeomFileUnits=cm  StepReaderType=HEX  ExportConvexHullGeometry=off  InertiaType=Custom  Mass=0.00030420054001085506  MassUnits=kg  CenterOfMass=[0.23057963245570592 -4.2158298307861626e-10 -1.6472469656016965e-11]  CenterOfMassUnits=cm  MomentsOfInertia=[3.0541038740142581e-06 2.6916548970402947e-05 2.6916548962268568e-05]  MomentsOfInertiaUnits=kg*cm^2  ProductsOfInertia=[0 0 0]  ProductsOfInertiaUnits=kg*cm^2  BasedOnType=Density  Density=1000  DensityUnits=kg/(m^3)  DoExposeReferenceFrame=on  SerializedFrames=<Frames/>  GraphicType=FromGeometry  MarkerShape=Sphere  MarkerSize=10  MarkerSizeUnits=m  GraphicVisPropType=SimpleVisualProperties  GraphicDiffuseColor=[0.72282352941176464 0.72282352941176464 0.72282352941176464]  GraphicSpecularColor=[0.5 0.5 0.5 1.0]  GraphicAmbientColor=[0.15 0.15 0.15 1.0]  GraphicEmissiveColor=[0.0 0.0 0.0 1.0]  GraphicShininess=75  GraphicOpacity=1
  F : PMIOPort  Side=Left
  connections:
  ReferenceFrame/RConn1 -- Solid/RConn1 -- F/RConn1

== system sm_import_stewart_platform/Stewart Platform/Imported Stewart Platform/ActuatorAssm1_2/CarrierAssm_1_RIGID/Recessed_Pan_Head_Screw_M2x8_48_Z_7_RIGID ==
  ReferenceFrame : sm_lib/Frames and Transforms/Reference Frame
  Solid : sm_lib/Body Elements/File Solid  ExtGeomFileName=Recessed_Pan_Head_Screw_M2x8_48_Z_Default_sldprt.STL  UnitType=Custom  ExtGeomFileUnits=cm  StepReaderType=HEX  ExportConvexHullGeometry=off  InertiaType=Custom  Mass=0.00030420054001085506  MassUnits=kg  CenterOfMass=[0.23057963245570592 -4.2158298307861626e-10 -1.6472469656016965e-11]  CenterOfMassUnits=cm  MomentsOfInertia=[3.0541038740142581e-06 2.6916548970402947e-05 2.6916548962268568e-05]  MomentsOfInertiaUnits=kg*cm^2  ProductsOfInertia=[0 0 0]  ProductsOfInertiaUnits=kg*cm^2  BasedOnType=Density  Density=1000  DensityUnits=kg/(m^3)  DoExposeReferenceFrame=on  SerializedFrames=<Frames/>  GraphicType=FromGeometry  MarkerShape=Sphere  MarkerSize=10  MarkerSizeUnits=m  GraphicVisPropType=SimpleVisualProperties  GraphicDiffuseColor=[0.72282352941176464 0.72282352941176464 0.72282352941176464]  GraphicSpecularColor=[0.5 0.5 0.5 1.0]  GraphicAmbientColor=[0.15 0.15 0.15 1.0]  GraphicEmissiveColor=[0.0 0.0 0.0 1.0]  GraphicShininess=75  GraphicOpacity=1
  F : PMIOPort  Side=Left
  connections:
  ReferenceFrame/RConn1 -- Solid/RConn1 -- F/RConn1

== system sm_import_stewart_platform/Stewart Platform/Imported Stewart Platform/ActuatorAssm1_2/CarrierAssm_1_RIGID/Recessed_Pan_Head_Screw_M2x8_48_Z_8_RIGID ==
  ReferenceFrame : sm_lib/Frames and Transforms/Reference Frame
  Solid : sm_lib/Body Elements/File Solid  ExtGeomFileName=Recessed_Pan_Head_Screw_M2x8_48_Z_Default_sldprt.STL  UnitType=Custom  ExtGeomFileUnits=cm  StepReaderType=HEX  ExportConvexHullGeometry=off  InertiaType=Custom  Mass=0.00030420054001085506  MassUnits=kg  CenterOfMass=[0.23057963245570592 -4.2158298307861626e-10 -1.6472469656016965e-11]  CenterOfMassUnits=cm  MomentsOfInertia=[3.0541038740142581e-06 2.6916548970402947e-05 2.6916548962268568e-05]  MomentsOfInertiaUnits=kg*cm^2  ProductsOfInertia=[0 0 0]  ProductsOfInertiaUnits=kg*cm^2  BasedOnType=Density  Density=1000  DensityUnits=kg/(m^3)  DoExposeReferenceFrame=on  SerializedFrames=<Frames/>  GraphicType=FromGeometry  MarkerShape=Sphere  MarkerSize=10  MarkerSizeUnits=m  GraphicVisPropType=SimpleVisualProperties  GraphicDiffuseColor=[0.72282352941176464 0.72282352941176464 0.72282352941176464]  GraphicSpecularColor=[0.5 0.5 0.5 1.0]  GraphicAmbientColor=[0.15 0.15 0.15 1.0]  GraphicEmissiveColor=[0.0 0.0 0.0 1.0]  GraphicShininess=75  GraphicOpacity=1
  F : PMIOPort  Side=Left
  connections:
  ReferenceFrame/RConn1 -- Solid/RConn1 -- F/RConn1

== system sm_import_stewart_platform/Stewart Platform/Imported Stewart Platform/ActuatorAssm1_2/CarrierAssm_1_RIGID/Recessed_Pan_Head_Screw_M2x8_48_Z_9_RIGID ==
  ReferenceFrame : sm_lib/Frames and Transforms/Reference Frame
  Solid : sm_lib/Body Elements/File Solid  ExtGeomFileName=Recessed_Pan_Head_Screw_M2x8_48_Z_Default_sldprt.STL  UnitType=Custom  ExtGeomFileUnits=cm  StepReaderType=HEX  ExportConvexHullGeometry=off  InertiaType=Custom  Mass=0.00030420054001085506  MassUnits=kg  CenterOfMass=[0.23057963245570592 -4.2158298307861626e-10 -1.6472469656016965e-11]  CenterOfMassUnits=cm  MomentsOfInertia=[3.0541038740142581e-06 2.6916548970402947e-05 2.6916548962268568e-05]  MomentsOfInertiaUnits=kg*cm^2  ProductsOfInertia=[0 0 0]  ProductsOfInertiaUnits=kg*cm^2  BasedOnType=Density  Density=1000  DensityUnits=kg/(m^3)  DoExposeReferenceFrame=on  SerializedFrames=<Frames/>  GraphicType=FromGeometry  MarkerShape=Sphere  MarkerSize=10  MarkerSizeUnits=m  GraphicVisPropType=SimpleVisualProperties  GraphicDiffuseColor=[0.72282352941176464 0.72282352941176464 0.72282352941176464]  GraphicSpecularColor=[0.5 0.5 0.5 1.0]  GraphicAmbientColor=[0.15 0.15 0.15 1.0]  GraphicEmissiveColor=[0.0 0.0 0.0 1.0]  GraphicShininess=75  GraphicOpacity=1
  F : PMIOPort  Side=Left
  connections:
  ReferenceFrame/RConn1 -- Solid/RConn1 -- F/RConn1

== system sm_import_stewart_platform/Stewart Platform/Imported Stewart Platform/ActuatorAssm1_2/CarrierAssm_1_RIGID/RenishawMount_1_RIGID ==
  ReferenceFrame : sm_lib/Frames and Transforms/Reference Frame
  Solid : sm_lib/Body Elements/File Solid  ExtGeomFileName=RenishawMount_Default_sldprt.STL  UnitType=Custom  ExtGeomFileUnits=cm  StepReaderType=HEX  ExportConvexHullGeometry=off  InertiaType=Custom  Mass=0.0034829489745196911  MassUnits=kg  CenterOfMass=[-0.48366741360957877 1.1533475803521882 1.7986253563001275]  CenterOfMassUnits=cm  MomentsOfInertia=[0.0021256933436925264 0.0030334445570311102 0.0012018141009422806]  MomentsOfInertiaUnits=kg*cm^2  ProductsOfInertia=[-3.2141879326220469e-05 -0.00044181135531947503 -5.1856038445014919e-05]  ProductsOfInertiaUnits=kg*cm^2  BasedOnType=Density  Density=1000  DensityUnits=kg/(m^3)  DoExposeReferenceFrame=on  SerializedFrames=<Frames/>  GraphicType=FromGeometry  MarkerShape=Sphere  MarkerSize=10  MarkerSizeUnits=m  GraphicVisPropType=SimpleVisualProperties  GraphicDiffuseColor=[0.48188235294117643 0 0.48188235294117643]  GraphicSpecularColor=[0.5 0.5 0.5 1.0]  GraphicAmbientColor=[0.15 0.15 0.15 1.0]  GraphicEmissiveColor=[0.0 0.0 0.0 1.0]  GraphicShininess=75  GraphicOpacity=1
  F : PMIOPort  Side=Left
  connections:
  ReferenceFrame/RConn1 -- Solid/RConn1 -- F/RConn1

== system sm_import_stewart_platform/Stewart Platform/Imported Stewart Platform/ActuatorAssm1_2/CarrierAssm_1_RIGID/SV2075_1_RIGID ==
  ReferenceFrame : sm_lib/Frames and Transforms/Reference Frame
  Solid : sm_lib/Body Elements/File Solid  ExtGeomFileName=SV2075_Default_sldprt.STL  UnitType=Custom  ExtGeomFileUnits=cm  StepReaderType=HEX  ExportConvexHullGeometry=off  InertiaType=Custom  Mass=0.0058459106101348196  MassUnits=kg  CenterOfMass=[-0.3298949175327261 0.0096923486215533452 3.75]  CenterOfMassUnits=cm  MomentsOfInertia=[0.027698839272727555 0.027673933267832958 0.00032822959311509738]  MomentsOfInertiaUnits=kg*cm^2  ProductsOfInertia=[0 0 1.1416492577499715e-06]  ProductsOfInertiaUnits=kg*cm^2  BasedOnType=Density  Density=1000  DensityUnits=kg/(m^3)  DoExposeReferenceFrame=on  SerializedFrames=<Frames/>  GraphicType=FromGeometry  MarkerShape=Sphere  MarkerSize=10  MarkerSizeUnits=m  GraphicVisPropType=SimpleVisualProperties  GraphicDiffuseColor=[0.97999999999999998 0.97999999999999998 0.97999999999999998]  GraphicSpecularColor=[0.5 0.5 0.5 1.0]  GraphicAmbientColor=[0.15 0.15 0.15 1.0]  GraphicEmissiveColor=[0.0 0.0 0.0 1.0]  GraphicShininess=75  GraphicOpacity=1
  F : PMIOPort  Side=Left
  connections:
  ReferenceFrame/RConn1 -- Solid/RConn1 -- F/RConn1

== system sm_import_stewart_platform/Stewart Platform/Imported Stewart Platform/ActuatorAssm1_2/CarrierAssm_1_RIGID/SV2075_2_RIGID ==
  ReferenceFrame : sm_lib/Frames and Transforms/Reference Frame
  Solid : sm_lib/Body Elements/File Solid  ExtGeomFileName=SV2075_Default_sldprt.STL  UnitType=Custom  ExtGeomFileUnits=cm  StepReaderType=HEX  ExportConvexHullGeometry=off  InertiaType=Custom  Mass=0.0058459106101348196  MassUnits=kg  CenterOfMass=[-0.3298949175327261 0.0096923486215533452 3.75]  CenterOfMassUnits=cm  MomentsOfInertia=[0.027698839272727555 0.027673933267832958 0.00032822959311509738]  MomentsOfInertiaUnits=kg*cm^2  ProductsOfInertia=[0 0 1.1416492577499715e-06]  ProductsOfInertiaUnits=kg*cm^2  BasedOnType=Density  Density=1000  DensityUnits=kg/(m^3)  DoExposeReferenceFrame=on  SerializedFrames=<Frames/>  GraphicType=FromGeometry  MarkerShape=Sphere  MarkerSize=10  MarkerSizeUnits=m  GraphicVisPropType=SimpleVisualProperties  GraphicDiffuseColor=[0.97999999999999998 0.97999999999999998 0.97999999999999998]  GraphicSpecularColor=[0.5 0.5 0.5 1.0]  GraphicAmbientColor=[0.15 0.15 0.15 1.0]  GraphicEmissiveColor=[0.0 0.0 0.0 1.0]  GraphicShininess=75  GraphicOpacity=1
  F : PMIOPort  Side=Left
  connections:
  ReferenceFrame/RConn1 -- Solid/RConn1 -- F/RConn1

== system sm_import_stewart_platform/Stewart Platform/Imported Stewart Platform/ActuatorAssm1_2/CarrierAssm_1_RIGID/ShaftStop_1_RIGID ==
  ReferenceFrame : sm_lib/Frames and Transforms/Reference Frame
  Solid : sm_lib/Body Elements/File Solid  ExtGeomFileName=ShaftStop_Default_sldprt.STL  UnitType=Custom  ExtGeomFileUnits=cm  StepReaderType=HEX  ExportConvexHullGeometry=off  InertiaType=Custom  Mass=0.005469591348952421  MassUnits=kg  CenterOfMass=[0.027829313128910391 0.38961039839964368 1.7949999999714594]  CenterOfMassUnits=cm  MomentsOfInertia=[0.0058998318849362956 0.0058998318849362956 0.0001702498370075098]  MomentsOfInertiaUnits=kg*cm^2  ProductsOfInertia=[0 0 0]  ProductsOfInertiaUnits=kg*cm^2  BasedOnType=Density  Density=1000  DensityUnits=kg/(m^3)  DoExposeReferenceFrame=on  SerializedFrames=<Frames/>  GraphicType=FromGeometry  MarkerShape=Sphere  MarkerSize=10  MarkerSizeUnits=m  GraphicVisPropType=SimpleVisualProperties  GraphicDiffuseColor=[0.95999999999999996 0.57599999999999996 0.95999999999999996]  GraphicSpecularColor=[0.5 0.5 0.5 1.0]  GraphicAmbientColor=[0.15 0.15 0.15 1.0]  GraphicEmissiveColor=[0.0 0.0 0.0 1.0]  GraphicShininess=75  GraphicOpacity=1
  F : PMIOPort  Side=Left
  connections:
  ReferenceFrame/RConn1 -- Solid/RConn1 -- F/RConn1

== system sm_import_stewart_platform/Stewart Platform/Imported Stewart Platform/ActuatorAssm1_2/CarrierAssm_1_RIGID/Yoke_1_RIGID ==
  ReferenceFrame : sm_lib/Frames and Transforms/Reference Frame
  Solid : sm_lib/Body Elements/File Solid  ExtGeomFileName=Yoke_Default_sldprt.STL  UnitType=Custom  ExtGeomFileUnits=m  StepReaderType=HEX  ExportConvexHullGeometry=off  InertiaType=Custom  Mass=0.0085668068985893069  MassUnits=kg  CenterOfMass=[3.3036113322449594e-09 4.5392080360257641e-09 0.013809135161090778]  CenterOfMassUnits=m  MomentsOfInertia=[3.6198630707133227e-07 3.7260728672028368e-07 1.1777278033424778e-07]  MomentsOfInertiaUnits=kg*m^2  ProductsOfInertia=[1.5891854780888145e-13 3.9281797530062808e-13 -1.9646780999777998e-13]  ProductsOfInertiaUnits=kg*m^2  BasedOnType=Density  Density=1000  DensityUnits=kg/(m^3)  DoExposeReferenceFrame=on  SerializedFrames=<Frames/>  GraphicType=FromGeometry  MarkerShape=Sphere  MarkerSize=10  MarkerSizeUnits=m  GraphicVisPropType=SimpleVisualProperties  GraphicDiffuseColor=[0.77647058823529413 0.75686274509803919 0.73725490196078436]  GraphicSpecularColor=[0.5 0.5 0.5 1.0]  GraphicAmbientColor=[0.15 0.15 0.15 1.0]  GraphicEmissiveColor=[0.0 0.0 0.0 1.0]  GraphicShininess=75  GraphicOpacity=1
  F : PMIOPort  Side=Left
  connections:
  ReferenceFrame/RConn1 -- Solid/RConn1 -- F/RConn1

== system sm_import_stewart_platform/Stewart Platform/Imported Stewart Platform/ActuatorAssm1_2/DrivenAssm_1_RIGID/AI_F100128_1_RIGID ==
  ReferenceFrame : sm_lib/Frames and Transforms/Reference Frame
  Solid : sm_lib/Body Elements/File Solid  ExtGeomFileName=AI_F100128_Default_sldprt.STL  UnitType=Custom  ExtGeomFileUnits=cm  StepReaderType=HEX  ExportConvexHullGeometry=off  InertiaType=Custom  Mass=0.0040299565156394811  MassUnits=kg  CenterOfMass=[-0.49905837297776268 0.96045195055630594 1.3249999999926647]  CenterOfMassUnits=cm  MomentsOfInertia=[0.0023888072647819153 0.0023888072647819153 0.00012526124846764931]  MomentsOfInertiaUnits=kg*cm^2  ProductsOfInertia=[0 0 0]  ProductsOfInertiaUnits=kg*cm^2  BasedOnType=Density  Density=1000  DensityUnits=kg/(m^3)  DoExposeReferenceFrame=on  SerializedFrames=<Frames/>  GraphicType=FromGeometry  MarkerShape=Sphere  MarkerSize=10  MarkerSizeUnits=m  GraphicVisPropType=SimpleVisualProperties  GraphicDiffuseColor=[0.74917647058823522 0.71529411764705886 0.62117647058823533]  GraphicSpecularColor=[0.5 0.5 0.5 1.0]  GraphicAmbientColor=[0.15 0.15 0.15 1.0]  GraphicEmissiveColor=[0.0 0.0 0.0 1.0]  GraphicShininess=75  GraphicOpacity=1
  F : PMIOPort  Side=Left
  connections:
  ReferenceFrame/RConn1 -- Solid/RConn1 -- F/RConn1

== system sm_import_stewart_platform/Stewart Platform/Imported Stewart Platform/ActuatorAssm1_2/DrivenAssm_1_RIGID/CenterBlock_1_RIGID ==
  ReferenceFrame : sm_lib/Frames and Transforms/Reference Frame
  Solid : sm_lib/Body Elements/File Solid  ExtGeomFileName=CenterBlock_Default_sldprt.STL  UnitType=Custom  ExtGeomFileUnits=m  StepReaderType=HEX  ExportConvexHullGeometry=off  InertiaType=Custom  Mass=0.15488060929368022  MassUnits=kg  CenterOfMass=[3.9702492273162504e-10 0.0085548453484078982 0.0073903409320849722]  CenterOfMassUnits=m  MomentsOfInertia=[0.00010890652503703371 0.00010444238201152375 9.5940475818836812e-06]  MomentsOfInertiaUnits=kg*m^2  ProductsOfInertia=[4.2158985322383779e-06 -2.1448350722557156e-12 -1.0080769576195953e-13]  ProductsOfInertiaUnits=kg*m^2  BasedOnType=Density  Density=1000  DensityUnits=kg/(m^3)  DoExposeReferenceFrame=on  SerializedFrames=<Frames/>  GraphicType=FromGeometry  MarkerShape=Sphere  MarkerSize=10  MarkerSizeUnits=m  GraphicVisPropType=SimpleVisualProperties  GraphicDiffuseColor=[0 0 0]  GraphicSpecularColor=[0.5 0.5 0.5 1.0]  GraphicAmbientColor=[0.15 0.15 0.15 1.0]  GraphicEmissiveColor=[0.0 0.0 0.0 1.0]  GraphicShininess=75  GraphicOpacity=1
  F : PMIOPort  Side=Left
  connections:
  ReferenceFrame/RConn1 -- Solid/RConn1 -- F/RConn1

== system sm_import_stewart_platform/Stewart Platform/Imported Stewart Platform/ActuatorAssm1_2/DrivenAssm_1_RIGID/CeramicStrip5010_1_RIGID ==
  ReferenceFrame : sm_lib/Frames and Transforms/Reference Frame
  Solid : sm_lib/Body Elements/File Solid  ExtGeomFileName=CeramicStrip5010_Default_sldprt.STL  UnitType=Custom  ExtGeomFileUnits=cm  StepReaderType=HEX  ExportConvexHullGeometry=off  InertiaType=Custom  Mass=0.0012937499999999978  MassUnits=kg  CenterOfMass=[-0.47402595951185544 0.93613171356507663 0]  CenterOfMassUnits=cm  MomentsOfInertia=[0.006066878906249993 0.0061722656249999933 0.00011023828124999996]  MomentsOfInertiaUnits=kg*cm^2  ProductsOfInertia=[0 0 0]  ProductsOfInertiaUnits=kg*cm^2  BasedOnType=Density  Density=1000  DensityUnits=kg/(m^3)  DoExposeReferenceFrame=on  SerializedFrames=<Frames/>  GraphicType=FromGeometry  MarkerShape=Sphere  MarkerSize=10  MarkerSizeUnits=m  GraphicVisPropType=SimpleVisualProperties  GraphicDiffuseColor=[0.95999999999999996 0.95999999999999996 0.95999999999999996]  GraphicSpecularColor=[0.5 0.5 0.5 1.0]  GraphicAmbientColor=[0.15 0.15 0.15 1.0]  GraphicEmissiveColor=[0.0 0.0 0.0 1.0]  GraphicShininess=75  GraphicOpacity=1
  F : PMIOPort  Side=Left
  connections:
  ReferenceFrame/RConn1 -- Solid/RConn1 -- F/RConn1
